simulink model "frmBuilder_sl_interactions_with_sfun"  (R2017b)
settings: Solver=FixedStepAuto  StartTime=0.0  StopTime=10.0  RelTol=1e-3  EnableMultiTasking=on
undefined symbols (not defined in the file or in its folder): params
libraries: simulink x2
settings Model: NumberOfSteps=10  Creator=na364  LastModifiedBy=na364
settings DataIOCC: LimitDataPoints=on
settings OptimizationCC: LifeSpan=inf
settings DebuggingCC: AllowSymbolicDim=off  SFUnexpectedBacktrackingDiag=warning  SFNoUnconditionalDefaultTransitionDiag=warning  SFExecutionAtInitializationDiag=none
settings ModelReferenceCC: ModelReferenceNumInstancesAllowed=Single  PropagateSignalLabelsOutOfModel=off
settings CodeAppCC: StateflowObjectComments=on
settings GRTTargetCC: TargetLangStandard=C89/C90 (ANSI)
settings ConfigComp: CovMetricSettings=dw  CovHtmlReporting=on  CovSaveCumulativeToWorkspaceVar=on  CovSaveSingleToWorkspaceVar=on  CovExternalEMLEnable=off

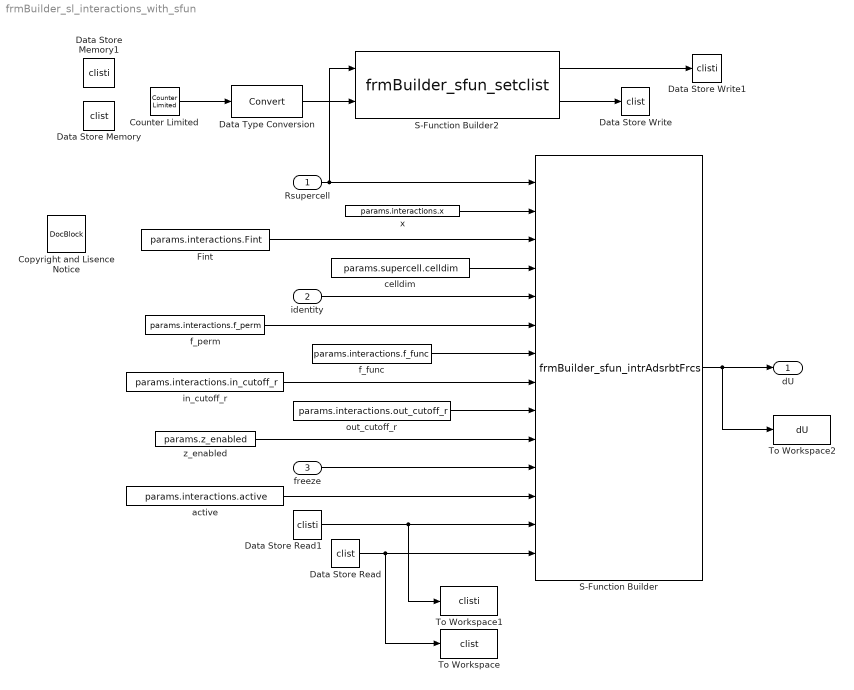
== system frmBuilder_sl_interactions_with_sfun ==
  Rsupercell : Inport  PortDimensions=[params.model_dim,sum([params.prtcl(:).Nprtcl])]
  identity : Inport  Port=2  PortDimensions=[1,sum([params.prtcl(:).Nprtcl])]
  freeze : Inport  Port=3  PortDimensions=[1,sum([params.prtcl(:).Nprtcl])]
  Copyright and Lisence Notice : simulink/Model-Wide Utilities/DocBlock  DocumentType=Text
      content=|
      | % Copyright (c) 2018, Nadav Avidor.
      | % All rights reserved.
      | % This file is part of the PIGLE - Particles Interacting in Generalized Langevin Equation simulator, subject to the
      | % GNU/GPL-3.0-or-later.
  Counter Limited : simulink/Sources/Counter Limited  uplimit=params.nclist-1  tsamp=-1
  Data Store Memory : DataStoreMemory  DataStoreName=clist  ReadBeforeWriteMsg=warning  WriteAfterWriteMsg=warning  WriteAfterReadMsg=warning  InitialValue=zeros(sum([params.prtcl(:).Nprtcl]),sum([params.prtcl(:).Nprtcl]))  ShowAdditionalParam=off  OutDataTypeStr=int32
  Data Store Memory1 : DataStoreMemory  DataStoreName=clisti  ReadBeforeWriteMsg=warning  WriteAfterWriteMsg=warning  WriteAfterReadMsg=warning  InitialValue=zeros(sum([params.prtcl(:).Nprtcl]),1)  ShowAdditionalParam=off  OutDataTypeStr=int32
  Data Store Read : DataStoreRead  DataStoreName=clist
  Data Store Read1 : DataStoreRead  DataStoreName=clisti
  Data Store Write : DataStoreWrite  DataStoreName=clist
  Data Store Write1 : DataStoreWrite  DataStoreName=clisti
  Data Type Conversion : DataTypeConversion
  Fint : Constant  Value=params.interactions.Fint
  S-Function Builder : S-Function  InitFcn=try, set_param(gcb,'FunctionName','frmBuilder_sfun_intrAdsrbtFrcs'), end  FunctionName=frmBuilder_sfun_intrAdsrbtFrcs  Parameters=sum([params.prtcl(:).Nprtcl]),size(params.interactions.Fint),params.model_dim  SFunctionModules=frmBuilder_sfun_intrAdsrbtFrcs_wrapper intrAdsrbtFrcs interp1lin  SFunctionDeploymentMode=off  EnableBusSupport=off  mask(S-Function Builder){}
      mask help: Simulink:masks:SFunctionBuilder_MD
      mask init:
      | val = [[.9  0.75 0.75 1 1 .9 .9 1]',[1 1 0.75 0.75 .9 .9 1 .9]'];try , sys = get_param(gcb,'SfunBuilderFcnName');if isempty(sys), sys = get_param(gcb,'FunctionName'); end,catch, sys = get_param(gcb,'FunctionName'); end
      settings: CopyFcn=set_param(gcbh,'LinkStatus','none')  PreSaveFcn=try, set_param(gcb,'FunctionName','frmBuilder_sfun_intrAdsrbtFrcs'), end  OpenFcn=sfunctionwizard(gcbh)
      mask Display: plot(val(:,1),val(:,2)),disp(sys), port_label('input',1,'pos'), port_label('input',2,'x'), port_label('input',3,'fTbltd'), port_label('input',4,'celldim'), port_label('input',5,'identity'), port_label('input',6,'f_perm'), port_label('input',7,'f_func'), port_label('input',8,'in_cutoff_r'), port_label('input',9,'out_cutoff_r'), port_label('input',10,'z_enabled'), port_label('input',11,'freeze'), port_label('input',12,'active'), port_label('input',13,'clisti'), port_label('input',14,'clist'), port_label('output',1,'iaf')
  S-Function Builder2 : S-Function  InitFcn=try, set_param(gcb,'FunctionName','frmBuilder_sfun_setclist'), end  FunctionName=frmBuilder_sfun_setclist  Parameters=params.supercell.celldim,params.interactions.out_cutoff_r  SFunctionModules=frmBuilder_sfun_setclist_wrapper setclist  SFunctionDeploymentMode=off  EnableBusSupport=off  mask(S-Function Builder){}
      mask help: Simulink:masks:SFunctionBuilder_MD
      mask init: same as frmBuilder_sl_interactions_with_sfun/S-Function Builder
      settings: CopyFcn=set_param(gcbh,'LinkStatus','none')  PreSaveFcn=try, set_param(gcb,'FunctionName','frmBuilder_sfun_setclist'), end  OpenFcn=sfunctionwizard(gcbh)
      mask Display: plot(val(:,1),val(:,2)),disp(sys), port_label('input',1,'pos'), port_label('input',2,'calc_clist'), port_label('output',1,'clisti'), port_label('output',2,'clist')
  To Workspace : ToWorkspace  VariableName=clist  SampleTime=-1
  To Workspace1 : ToWorkspace  VariableName=clisti  SampleTime=-1
  To Workspace2 : ToWorkspace  VariableName=dU  SampleTime=-1
      settings: Decimation=params.decimation
  active : Constant  Value=params.interactions.active
  celldim : Constant  Value=params.supercell.celldim
  f_func : Constant  Value=params.interactions.f_func
  f_perm : Constant  Value=params.interactions.f_perm
  in_cutoff_r : Constant  Value=params.interactions.in_cutoff_r
  out_cutoff_r : Constant  Value=params.interactions.out_cutoff_r
  x : Constant  Value=params.interactions.x
  z_enabled : Constant  Value=params.z_enabled
  dU : Outport  PortDimensions=[params.model_dim,params.Nprtcl]
  wires:
  Rsupercell/1 -> S-Function Builder2/1, S-Function Builder/1
  celldim/1 -> S-Function Builder/4
  Fint/1 -> S-Function Builder/3
  x/1 -> S-Function Builder/2
  identity/1 -> S-Function Builder/5
  f_perm/1 -> S-Function Builder/6
  f_func/1 -> S-Function Builder/7
  in_cutoff_r/1 -> S-Function Builder/8
  out_cutoff_r/1 -> S-Function Builder/9
  z_enabled/1 -> S-Function Builder/10
  S-Function Builder/1 -> To Workspace2/1, dU/1
  freeze/1 -> S-Function Builder/11
  active/1 -> S-Function Builder/12
  Data Store Read1/1 -> S-Function Builder/13, To Workspace1/1
  Data Store Read/1 -> To Workspace/1, S-Function Builder/14
  S-Function Builder2/2 -> Data Store Write/1
  S-Function Builder2/1 -> Data Store Write1/1
  Counter Limited/1 -> Data Type Conversion/1
  Data Type Conversion/1 -> S-Function Builder2/2
